simulink model "PFC_dq_2019_frequentielle"  (R2023a)
settings: Solver=VariableStepAuto  StartTime=0.0  StopTime=temp_simu  RelTol=Te/20
undefined symbols (not defined in the file): C, Control_Udc, i_de, id_sat, L, r, R_K_PIDf, Rch, Te, Ud, Udc_cons, Uq, w
libraries: cstblocks x2
settings Model: Creator=xshi  LastModifiedBy=dougl
settings SolverCC: AlgebraicLoopSolver=TrustRegion
settings DebuggingCC: AlgebraicLoopMsg=none  UnconnectedInputMsg=warning  UnconnectedOutputMsg=warning  UnconnectedLineMsg=warning
settings ModelReferenceCC: EnableRefExpFcnMdlSchedulingChecks=on
settings SFSimCC: CustomCodeUndefinedFunction=UseInterfaceOnly

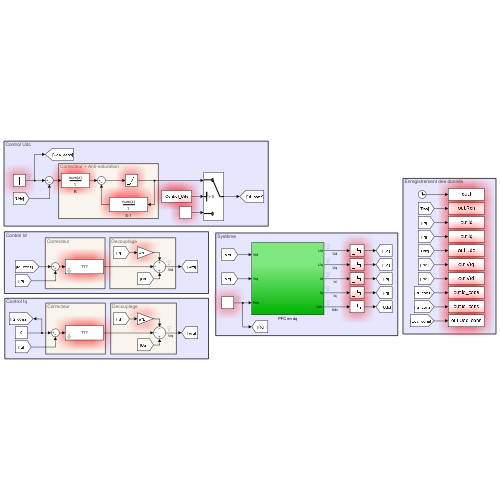
[thumbnail: Simulink's stored preview of the top-level diagram]
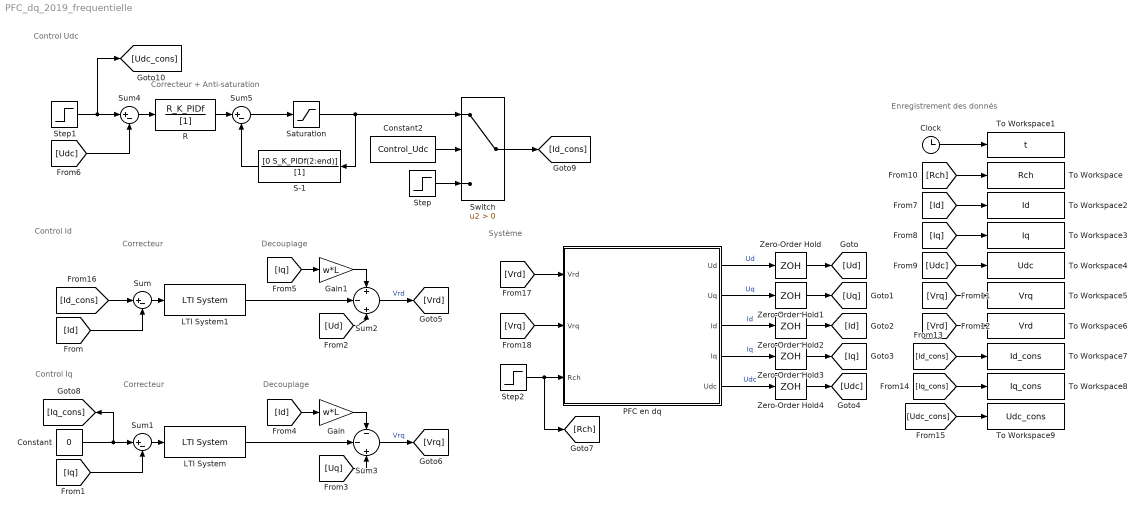
== system PFC_dq_2019_frequentielle ==
  note: Enregistrement des donnés
  note: Système
  note: Decouplage
  note: Control Iq
  note: Control Id
  note: Control Udc
  note: Decouplage
  note: Correcteur + Anti-saturation
  note: Correcteur
  note: Correcteur
  Clock : Clock
  Constant : Constant  Value=0  SampleTime=-1
  Constant2 : Constant  Value=Control_Udc
  Gain : Gain  Gain=w*L
  Gain1 : Gain  Gain=w*L
  LTI System : cstblocks/LTI System  sys=K_PI  IC=[]
  LTI System1 : cstblocks/LTI System  sys=K_PI  IC=[]
  PFC en dq : Subsystem
  R : DiscreteFilter  Numerator=R_K_PIDf  Denominator=[1]  SampleTime=Te
  S-1 : DiscreteFilter  Numerator=[0 S_K_PIDf(2:end)]  Denominator=[1]  SampleTime=Te
  Saturation : Saturate  UpperLimit=id_sat  LowerLimit=-id_sat
  Step : Step  Before=i_de  After=i_de/2  SampleTime=0
  Step1 : Step  Time=0  After=Udc_cons  SampleTime=0
  Step2 : Step  Time=3  Before=Rch  After=Rch/2  SampleTime=0
  Sum{,1,4..5} (4 alike) : Sum  Inputs=|+-
  Sum2 : Sum  Inputs=+|-|+
  Sum3 : Sum  Inputs=-|-|+
  Switch : Switch  Criteria=u2 > Threshold  SaturateOnIntegerOverflow=off  InputSameDT=off
  To Workspace : ToWorkspace  VariableName=Rch  SampleTime=Te
  To Workspace1 : ToWorkspace  VariableName=t  SampleTime=Te
  To Workspace2 : ToWorkspace  VariableName=Id  SampleTime=Te
  To Workspace3 : ToWorkspace  VariableName=Iq  SampleTime=Te
  To Workspace4 : ToWorkspace  VariableName=Udc  SampleTime=Te
  To Workspace5 : ToWorkspace  VariableName=Vrq  SampleTime=Te
  To Workspace6 : ToWorkspace  VariableName=Vrd  SampleTime=Te
  To Workspace7 : ToWorkspace  VariableName=Id_cons  SampleTime=Te
  To Workspace8 : ToWorkspace  VariableName=Iq_cons  SampleTime=Te
  To Workspace9 : ToWorkspace  VariableName=Udc_cons  SampleTime=Te
  Zero-Order Hold{,1..4} (5 alike) : ZeroOrderHold  SampleTime=Te
  wires:
  Sum1/1 -> LTI System/1
  PFC en dq/1(Ud) -> Zero-Order Hold/1  "Ud"
  PFC en dq/2(Uq) -> Zero-Order Hold1/1  "Uq"
  PFC en dq/3(Id) -> Zero-Order Hold2/1  "Id"
  PFC en dq/4(Iq) -> Zero-Order Hold3/1  "Iq"
  PFC en dq/5(Udc) -> Zero-Order Hold4/1  "Udc"
  [Id] -> Sum/2
  Sum/1 -> LTI System1/1
  [Iq] -> Sum1/2
  LTI System1/1 -> Sum2/2
  LTI System/1 -> Sum3/2
  [Ud] -> Sum2/3
  [Uq] -> Sum3/3
  [Id] -> Gain/1
  Gain/1 -> Sum3/1
  [Iq] -> Gain1/1
  Constant/1 -> Sum1/1, [Iq_cons]
  Gain1/1 -> Sum2/1
  Sum2/1 -> [Vrd]  "Vrd"
  Sum3/1 -> [Vrq]  "Vrq"
  Step2/1 -> [Rch], PFC en dq/3(Rch)
  Step1/1 -> [Udc_cons], Sum4/1
  [Udc] -> Sum4/2
  Sum4/1 -> R/1
  Step/1 -> Switch/3
  Constant2/1 -> Switch/2
  [Rch] -> To Workspace/1
  Clock/1 -> To Workspace1/1
  [Id] -> To Workspace2/1
  [Iq] -> To Workspace3/1
  [Udc] -> To Workspace4/1
  [Vrq] -> To Workspace5/1
  [Vrd] -> To Workspace6/1
  [Id_cons] -> To Workspace7/1
  [Iq_cons] -> To Workspace8/1
  [Udc_cons] -> To Workspace9/1
  Sum5/1 -> Saturation/1
  R/1 -> Sum5/1
  S-1/1 -> Sum5/2
  Saturation/1 -> Switch/1, S-1/1
  Zero-Order Hold/1 -> [Ud]
  Zero-Order Hold1/1 -> [Uq]
  Zero-Order Hold2/1 -> [Id]
  Zero-Order Hold3/1 -> [Iq]
  Zero-Order Hold4/1 -> [Udc]
  Switch/1 -> [Id_cons]
  [Id_cons] -> Sum/1
  [Vrd] -> PFC en dq/1(Vrd)
  [Vrq] -> PFC en dq/2(Vrq)

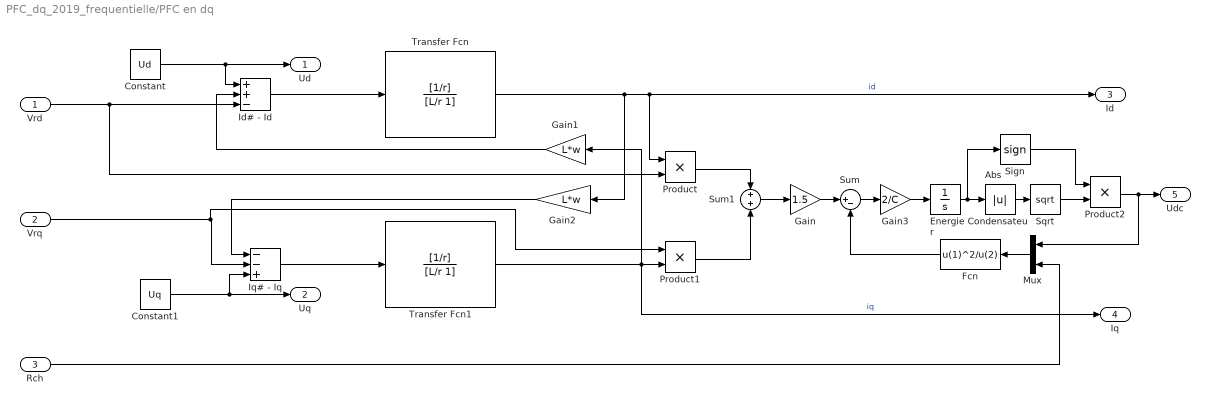
== system PFC_dq_2019_frequentielle/PFC en dq ==
  Vrd : Inport
  Vrq : Inport  Port=2
  Rch : Inport  Port=3
  Abs : Abs  SaturateOnIntegerOverflow=off
  Constant : Constant  Value=Ud
  Constant1 : Constant  Value=Uq
  Energie Condensateur : Integrator  InitialCondition=400^2
  Fcn : Fcn  Expr=u(1)^2/u(2)
  Gain : Gain  Gain=1.5
  Gain1 : Gain  Gain=L*w
  Gain2 : Gain  Gain=L*w
  Gain3 : Gain  Gain=2/C
  Id# - Id : Sum  Inputs=++-  InputSameDT=on  SaturateOnIntegerOverflow=on  OutDataTypeStr=Inherit: Same as first input
  Iq# - Iq : Sum  Inputs=--+  InputSameDT=on  SaturateOnIntegerOverflow=on  OutDataTypeStr=Inherit: Same as first input
  Mux : Mux  Inputs=2
  Product : Product
  Product1 : Product
  Product2 : Product
  Sign : Signum
  Sqrt : Sqrt
  Sum : Sum  Inputs=|+-
  Sum1 : Sum
  Transfer Fcn : TransferFcn  Numerator=[1/r]  Denominator=[L/r 1]
  Transfer Fcn1 : TransferFcn  Numerator=[1/r]  Denominator=[L/r 1]
  Ud : Outport  VectorParamsAs1DForOutWhenUnconnected=off
  Uq : Outport  Port=2  VectorParamsAs1DForOutWhenUnconnected=off
  Id : Outport  Port=3  VectorParamsAs1DForOutWhenUnconnected=off
  Iq : Outport  Port=4  VectorParamsAs1DForOutWhenUnconnected=off
  Udc : Outport  Port=5  VectorParamsAs1DForOutWhenUnconnected=off
  wires:
  Mux/1 -> Fcn/1
  Fcn/1 -> Sum/2
  Gain/1 -> Sum/1
  Vrq/1 -> Product1/1, Iq# - Iq/2
  Rch/1 -> Mux/2
  Transfer Fcn1/1 -> Gain1/1, Product1/2, Iq/1  "iq"
  Gain1/1 -> Id# - Id/2
  Gain2/1 -> Iq# - Iq/1
  Id# - Id/1 -> Transfer Fcn/1
  Transfer Fcn/1 -> Product/1, Id/1, Gain2/1  "id"
  Vrd/1 -> Product/2, Id# - Id/3
  Constant/1 -> Ud/1, Id# - Id/1
  Iq# - Iq/1 -> Transfer Fcn1/1
  Constant1/1 -> Uq/1, Iq# - Iq/3
  Sum1/1 -> Gain/1
  Product/1 -> Sum1/1
  Product1/1 -> Sum1/2
  Product2/1 -> Mux/1, Udc/1
  Gain3/1 -> Energie Condensateur/1
  Abs/1 -> Sqrt/1
  Energie Condensateur/1 -> Sign/1, Abs/1
  Sqrt/1 -> Product2/2
  Sign/1 -> Product2/1
  Sum/1 -> Gain3/1
